simulink model "discretoSIMULINK_PI"  (Simulink 7.4)
settings: Solver=ode3  StartTime=0.0  StopTime=20  FixedStep=Ta  RelTol=1e-3
values from neighbouring files (symbols this model uses):
  denp = [1 -0.9654 0 -0.0810 0 0 0 0 0.2549 0 0 -0.1930 -0.0543 0.0565 0.1138 -0.1976 0.2538 -0.0892]    [controle.m]    (also in controle_6polos.m = [1 -0.1106 -0.2860 -0.4816 0.5898 -0.3666 0.2016])
  nump = [0 0 0 0.5441 0.4959 0 -0.3858 0 0 0 0 0 0 0 0 0 0 0]    [controle.m]    (also in controle_6polos.m = [0.0154 -0.1308 -0.3082 1.1892 1.6618 1.5483 0.2994])
  Ta = 0.1    [Identificacao.m]    (also in controle.m = 0.01; controle_6polos.m = 0.01)
undefined symbols (not defined in the file or in its folder): amplitude, Kd_PI, Ki_PI, Kp_PI, ruido_media, ruido_variancia, saturacao_max, saturacao_min
settings Model: Creator=Fabiano  LastModifiedBy=Fabiano
settings DataIOCC: SignalLoggingName=sigsOut
settings DebuggingCC: SaveWithParameterizedLinksMsg=none  SignalResolutionControl=TryResolveAllWithWarning  SolverPrmCheckMsg=none  MultiTaskDSMMsg=warning  MultiTaskCondExecSysMsg=none  StrictBusMsg=None
settings HardwareCC: TargetUnknown=on
settings RTWCC: IncludeERTFirstTime=on

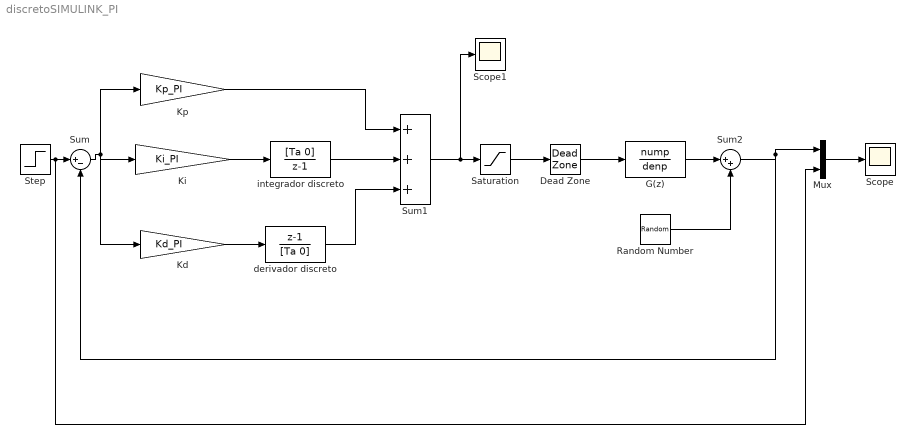
== system discretoSIMULINK_PI ==
  Dead Zone : DeadZone  LowerValue=banda_morta_ini  UpperValue=banda_morta_fim  SaturateOnIntegerOverflow=on
  G(z) : DiscreteTransferFcn  Numerator=nump  Denominator=denp  SampleTime=Ta
  Kd : Gain  Gain=Kd_PI  ParameterDataType=sfix(16)  ParameterScaling=2^0  OutDataType=sfix(16)  OutScaling=2^0  SaturateOnIntegerOverflow=on  OutDataTypeStr=Inherit: Same as input  ParamDataTypeStr=Inherit: Same as input
  Ki : Gain  Gain=Ki_PI  ParameterDataType=sfix(16)  ParameterScaling=2^0  OutDataType=sfix(16)  OutScaling=2^0  SaturateOnIntegerOverflow=on  OutDataTypeStr=Inherit: Same as input  ParamDataTypeStr=Inherit: Same as input
  Kp : Gain  Gain=Kp_PI  ParameterDataType=sfix(16)  ParameterScaling=2^0  OutDataType=sfix(16)  OutScaling=2^0  SaturateOnIntegerOverflow=on  OutDataTypeStr=Inherit: Same as input  ParamDataTypeStr=Inherit: Same as input
  Mux : Mux  Inputs=2
  Random Number : RandomNumber  Mean=ruido_media  Variance=ruido_variancia  SampleTime=0
  Saturation : Saturate  UpperLimit=saturacao_max  LowerLimit=saturacao_min
  Scope : Scope
      settings: TimeRange=10  SaveName=sinais  DataFormat=Array
  Scope1 : Scope
      settings: TimeRange=10  YMin=-1
  Step : Step  Time=0  After=amplitude  SampleTime=0
  Sum : Sum  Inputs=|+-  OutDataType=sfix(16)  OutScaling=2^0  SaturateOnIntegerOverflow=on
  Sum1 : Sum  Inputs=+++  OutDataType=sfix(16)  OutScaling=2^0  SaturateOnIntegerOverflow=on
  Sum2 : Sum  Inputs=|++  OutDataType=sfix(16)  OutScaling=2^0  SaturateOnIntegerOverflow=on
  derivador discreto : DiscreteTransferFcn  Numerator=[1 -1]  Denominator=[Ta 0]  SampleTime=Ta
  integrador discreto : DiscreteTransferFcn  Numerator=[Ta 0]  Denominator="[1  -1]"  SampleTime=Ta
  wires:
  Saturation/1 -> Dead Zone/1
  Step/1 -> Sum/1, Mux/2
  Kp/1 -> Sum1/1
  integrador discreto/1 -> Sum1/2
  Ki/1 -> integrador discreto/1
  Kd/1 -> derivador discreto/1
  Sum/1 -> Kp/1, Kd/1, Ki/1
  Sum1/1 -> Saturation/1, Scope1/1
  Mux/1 -> Scope/1
  G(z)/1 -> Sum2/1
  Random Number/1 -> Sum2/2
  Sum2/1 -> Mux/1, Sum/2
  derivador discreto/1 -> Sum1/3
  Dead Zone/1 -> G(z)/1
